simulink model "case8"  (R2024b)
settings: Solver=FixedStepAuto  StartTime=0  StopTime=1  FixedStep=1e-7  RelTol=1e-3
values from neighbouring files (symbols this model uses):
  SG_D_1_D = 0.01056    [IEEE9_case_parameters.m]    (also in case1_parameters.m; case2_parameters.m; case3_parameters.m; case4_parameters.m)
  SG_D_1_EnableSaturation = 0    [IEEE9_case_parameters.m]    (also in case1_parameters.m; case2_parameters.m; case3_parameters.m; case4_parameters.m)
  SG_D_1_f0 = 60    [IEEE9_case_parameters.m]    (also in case1_parameters.m; case2_parameters.m; case3_parameters.m; case4_parameters.m)
  SG_D_1_H = 7.5    [IEEE9_case_parameters.m]    (also in case1_parameters.m; case2_parameters.m; case3_parameters.m; case4_parameters.m)
  SG_D_1_K_A = 20    [IEEE9_case_parameters.m]    (also in case1_parameters.m; case2_parameters.m; case3_parameters.m; case4_parameters.m)
  SG_D_1_K_E = 1.000000e+1    (= 10)    [IEEE9_case_parameters.m]    (also in case1_parameters.m; case2_parameters.m; case3_parameters.m; case4_parameters.m)
  SG_D_1_K_F = 2.363    [IEEE9_case_parameters.m]    (also in case1_parameters.m; case2_parameters.m; case3_parameters.m; case4_parameters.m)
  SG_D_1_K_s = 0.5    [IEEE9_case_parameters.m]    (also in case1_parameters.m = 5; case2_parameters.m = 5; case3_parameters.m = 5; case4_parameters.m = 5)
  SG_D_1_R_a = 0.001088    [IEEE9_case_parameters.m]    (also in case1_parameters.m; case2_parameters.m; case3_parameters.m; case4_parameters.m)
  SG_D_1_S_A = 1    [IEEE9_case_parameters.m]    (also in case1_parameters.m; case2_parameters.m; case3_parameters.m; case4_parameters.m)
  SG_D_1_S_B = 0.103    [IEEE9_case_parameters.m]    (also in case1_parameters.m; case2_parameters.m; case3_parameters.m; case4_parameters.m)
  SG_D_1_S_N = 10.659857    [IEEE9_case_parameters.m]    (also in case1_parameters.m; case2_parameters.m; case3_parameters.m; case4_parameters.m)
  SG_D_1_SpeedPara = 200    [IEEE9_case_parameters.m]    (also in case1_parameters.m; case2_parameters.m; case3_parameters.m; case4_parameters.m)
  SG_D_1_T_0 = 0.720173    [IEEE9_case_parameters.m]    (also in case1_parameters.m = 0.755522; case2_parameters.m = 0.808931; case3_parameters.m = 0.869402; case4_parameters.m = 0.729316)
  SG_D_1_T_1 = 0.3    [IEEE9_case_parameters.m]    (also in case1_parameters.m; case2_parameters.m; case3_parameters.m; case4_parameters.m)
  SG_D_1_T_2 = 0.05    [IEEE9_case_parameters.m]    (also in case1_parameters.m; case2_parameters.m; case3_parameters.m; case4_parameters.m)
  SG_D_1_T_3 = 0.02    [IEEE9_case_parameters.m]    (also in case1_parameters.m; case2_parameters.m; case3_parameters.m; case4_parameters.m)
  SG_D_1_T_4 = 0.005    [IEEE9_case_parameters.m]    (also in case1_parameters.m; case2_parameters.m; case3_parameters.m; case4_parameters.m)
  SG_D_1_T_A = 0.02    [IEEE9_case_parameters.m]    (also in case1_parameters.m; case2_parameters.m; case3_parameters.m; case4_parameters.m)
  SG_D_1_T_dd = 8.000000e+0    (= 8)    [IEEE9_case_parameters.m]    (also in case1_parameters.m; case2_parameters.m; case3_parameters.m; case4_parameters.m)
  SG_D_1_T_ddd = 0.04    [IEEE9_case_parameters.m]    (also in case1_parameters.m; case2_parameters.m; case3_parameters.m; case4_parameters.m)
  SG_D_1_T_E = 0.314    [IEEE9_case_parameters.m]    (also in case1_parameters.m; case2_parameters.m; case3_parameters.m; case4_parameters.m)
  SG_D_1_T_F = 0.35    [IEEE9_case_parameters.m]    (also in case1_parameters.m; case2_parameters.m; case3_parameters.m; case4_parameters.m)
  SG_D_1_T_qd = 0.8    [IEEE9_case_parameters.m]    (also in case1_parameters.m; case2_parameters.m; case3_parameters.m; case4_parameters.m)
  SG_D_1_T_qdd = 0.02    [IEEE9_case_parameters.m]    (also in case1_parameters.m; case2_parameters.m; case3_parameters.m; case4_parameters.m)
  SG_D_1_T_speed = 0.1    [IEEE9_case_parameters.m]    (also in case1_parameters.m = 200; case2_parameters.m = 200; case3_parameters.m = 200; case4_parameters.m = 200)
  SG_D_1_T_w = 0.5    [IEEE9_case_parameters.m]    (also in case1_parameters.m; case2_parameters.m; case3_parameters.m; case4_parameters.m)
  SG_D_1_V_ref = 1.990276    [IEEE9_case_parameters.m]    (also in case1_parameters.m = 2.042296; case2_parameters.m = 2.051388; case3_parameters.m = 2.089584; case4_parameters.m = 2.01845)
  SG_D_1_w_ref = 376.991118    [IEEE9_case_parameters.m]    (also in case1_parameters.m; case2_parameters.m; case3_parameters.m; case4_parameters.m)
  SG_D_1_wb = 6.000000e+1    (= 60)    [IEEE9_case_parameters.m]    (also in case1_parameters.m; case2_parameters.m; case3_parameters.m; case4_parameters.m)
  SG_D_1_x_d = 1.9    [IEEE9_case_parameters.m]    (also in case1_parameters.m; case2_parameters.m; case3_parameters.m; case4_parameters.m)
  SG_D_1_x_dd = 0.302    [IEEE9_case_parameters.m]    (also in case1_parameters.m; case2_parameters.m; case3_parameters.m; case4_parameters.m)
  SG_D_1_x_ddd = 0.204    [IEEE9_case_parameters.m]    (also in case1_parameters.m; case2_parameters.m; case3_parameters.m; case4_parameters.m)
  SG_D_1_x_l = 0.05    [IEEE9_case_parameters.m]    (also in case1_parameters.m; case2_parameters.m; case3_parameters.m; case4_parameters.m)
  SG_D_1_x_q = 1.3    [IEEE9_case_parameters.m]    (also in case1_parameters.m; case2_parameters.m; case3_parameters.m; case4_parameters.m)
  SG_D_1_x_qd = 0.5    [IEEE9_case_parameters.m]    (also in case1_parameters.m; case2_parameters.m; case3_parameters.m; case4_parameters.m)
  SG_D_1_x_qdd = 0.3    [IEEE9_case_parameters.m]    (also in case1_parameters.m; case2_parameters.m; case3_parameters.m; case4_parameters.m)
  SG_D_2_D = 0.02    [IEEE9_case_parameters.m]    (also in case1_parameters.m; case2_parameters.m; case3_parameters.m; case4_parameters.m)
  SG_D_2_EnableSaturation = 0    [IEEE9_case_parameters.m]    (also in case1_parameters.m; case2_parameters.m; case3_parameters.m; case4_parameters.m)
  SG_D_2_f0 = 60    [IEEE9_case_parameters.m]    (also in case1_parameters.m; case2_parameters.m; case3_parameters.m; case4_parameters.m)
  SG_D_2_H = 8.000000e+0    (= 8)    [IEEE9_case_parameters.m]    (also in case1_parameters.m; case2_parameters.m; case3_parameters.m; case4_parameters.m)
  SG_D_2_K_A = 20    [IEEE9_case_parameters.m]    (also in case1_parameters.m; case2_parameters.m; case3_parameters.m; case4_parameters.m)
  SG_D_2_K_E = 1.000000e+1    (= 10)    [IEEE9_case_parameters.m]    (also in case1_parameters.m; case2_parameters.m; case3_parameters.m; case4_parameters.m)
  SG_D_2_K_F = 2.363    [IEEE9_case_parameters.m]    (also in case1_parameters.m; case2_parameters.m; case3_parameters.m; case4_parameters.m)
  SG_D_2_K_s = 0.5    [IEEE9_case_parameters.m]    (also in case1_parameters.m = 4; case2_parameters.m = 4; case3_parameters.m = 4; case4_parameters.m = 4)
  SG_D_2_R_a = 0.001088    [IEEE9_case_parameters.m]    (also in case1_parameters.m; case2_parameters.m; case3_parameters.m; case4_parameters.m)
  SG_D_2_S_A = 1    [IEEE9_case_parameters.m]    (also in case1_parameters.m; case2_parameters.m; case3_parameters.m; case4_parameters.m)
  SG_D_2_S_B = 0.103    [IEEE9_case_parameters.m]    (also in case1_parameters.m; case2_parameters.m; case3_parameters.m; case4_parameters.m)
  SG_D_2_S_N = 10.659857    [IEEE9_case_parameters.m]    (also in case1_parameters.m; case2_parameters.m; case3_parameters.m; case4_parameters.m)
  SG_D_2_SpeedPara = 200    [IEEE9_case_parameters.m]    (also in case1_parameters.m; case2_parameters.m; case3_parameters.m; case4_parameters.m)
  SG_D_2_T_0 = 1.632913    [IEEE9_case_parameters.m]    (also in case1_parameters.m = 1.632925; case2_parameters.m = 1.632915; case3_parameters.m = 1.632914; case4_parameters.m = 1.632927)
  SG_D_2_T_1 = 0.2    [IEEE9_case_parameters.m]    (also in case1_parameters.m; case2_parameters.m; case3_parameters.m; case4_parameters.m)
  SG_D_2_T_2 = 0.05    [IEEE9_case_parameters.m]    (also in case1_parameters.m; case2_parameters.m; case3_parameters.m; case4_parameters.m)
  SG_D_2_T_3 = 0.02    [IEEE9_case_parameters.m]    (also in case1_parameters.m; case2_parameters.m; case3_parameters.m; case4_parameters.m)
  SG_D_2_T_4 = 0.005    [IEEE9_case_parameters.m]    (also in case1_parameters.m; case2_parameters.m; case3_parameters.m; case4_parameters.m)
  SG_D_2_T_A = 0.02    [IEEE9_case_parameters.m]    (also in case1_parameters.m; case2_parameters.m; case3_parameters.m; case4_parameters.m)
  SG_D_2_T_dd = 7.9    [IEEE9_case_parameters.m]    (also in case1_parameters.m; case2_parameters.m; case3_parameters.m; case4_parameters.m)
  SG_D_2_T_ddd = 0.04    [IEEE9_case_parameters.m]    (also in case1_parameters.m; case2_parameters.m; case3_parameters.m; case4_parameters.m)
  SG_D_2_T_E = 0.314    [IEEE9_case_parameters.m]    (also in case1_parameters.m; case2_parameters.m; case3_parameters.m; case4_parameters.m)
  SG_D_2_T_F = 0.35    [IEEE9_case_parameters.m]    (also in case1_parameters.m; case2_parameters.m; case3_parameters.m; case4_parameters.m)
  SG_D_2_T_qd = 0.8    [IEEE9_case_parameters.m]    (also in case1_parameters.m; case2_parameters.m; case3_parameters.m; case4_parameters.m)
  SG_D_2_T_qdd = 0.015    [IEEE9_case_parameters.m]    (also in case1_parameters.m; case2_parameters.m; case3_parameters.m; case4_parameters.m)
  SG_D_2_T_speed = 0.1    [IEEE9_case_parameters.m]    (also in case1_parameters.m = 150; case2_parameters.m = 150; case3_parameters.m = 150; case4_parameters.m = 150)
  SG_D_2_T_w = 0.35    [IEEE9_case_parameters.m]    (also in case1_parameters.m; case2_parameters.m; case3_parameters.m; case4_parameters.m)
  SG_D_2_V_ref = 2.58547    [IEEE9_case_parameters.m]    (also in case1_parameters.m = 2.597896; case2_parameters.m = 2.587136; case3_parameters.m = 2.586042; case4_parameters.m = 2.599679)
  SG_D_2_w_ref = 376.991118    [IEEE9_case_parameters.m]    (also in case1_parameters.m; case2_parameters.m; case3_parameters.m; case4_parameters.m)
  SG_D_2_wb = 6.000000e+1    (= 60)    [IEEE9_case_parameters.m]    (also in case1_parameters.m; case2_parameters.m; case3_parameters.m; case4_parameters.m)
  SG_D_2_x_d = 1.8    [IEEE9_case_parameters.m]    (also in case1_parameters.m; case2_parameters.m; case3_parameters.m; case4_parameters.m)
  SG_D_2_x_dd = 0.302    [IEEE9_case_parameters.m]    (also in case1_parameters.m; case2_parameters.m; case3_parameters.m; case4_parameters.m)
  SG_D_2_x_ddd = 0.204    [IEEE9_case_parameters.m]    (also in case1_parameters.m; case2_parameters.m; case3_parameters.m; case4_parameters.m)
  SG_D_2_x_l = 0.05    [IEEE9_case_parameters.m]    (also in case1_parameters.m; case2_parameters.m; case3_parameters.m; case4_parameters.m)
  SG_D_2_x_q = 1.25    [IEEE9_case_parameters.m]    (also in case1_parameters.m; case2_parameters.m; case3_parameters.m; case4_parameters.m)
  SG_D_2_x_qd = 0.5    [IEEE9_case_parameters.m]    (also in case1_parameters.m; case2_parameters.m; case3_parameters.m; case4_parameters.m)
  SG_D_2_x_qdd = 0.3    [IEEE9_case_parameters.m]    (also in case1_parameters.m; case2_parameters.m; case3_parameters.m; case4_parameters.m)
  SG_D_3_D = 0.02    [IEEE9_case_parameters.m]    (also in case1_parameters.m; case2_parameters.m; case3_parameters.m; case4_parameters.m)
  SG_D_3_EnableSaturation = 0    [IEEE9_case_parameters.m]    (also in case1_parameters.m; case2_parameters.m; case3_parameters.m; case4_parameters.m)
  SG_D_3_f0 = 60    [IEEE9_case_parameters.m]    (also in case1_parameters.m; case2_parameters.m; case3_parameters.m; case4_parameters.m)
  SG_D_3_H = 7.7    [IEEE9_case_parameters.m]    (also in case1_parameters.m; case2_parameters.m; case3_parameters.m; case4_parameters.m)
  SG_D_3_K_A = 20    [IEEE9_case_parameters.m]    (also in case1_parameters.m; case2_parameters.m; case3_parameters.m; case4_parameters.m)
  SG_D_3_K_E = 1.000000e+1    (= 10)    [IEEE9_case_parameters.m]    (also in case1_parameters.m; case2_parameters.m; case3_parameters.m; case4_parameters.m)
  SG_D_3_K_F = 2.363    [IEEE9_case_parameters.m]    (also in case1_parameters.m; case2_parameters.m; case3_parameters.m; case4_parameters.m)
  SG_D_3_K_s = 0.2    [IEEE9_case_parameters.m]    (also in case1_parameters.m = 2; case2_parameters.m = 2; case3_parameters.m = 2; case4_parameters.m = 2)
  SG_D_3_R_a = 0.001088    [IEEE9_case_parameters.m]    (also in case1_parameters.m; case2_parameters.m; case3_parameters.m; case4_parameters.m)
  SG_D_3_S_A = 1    [IEEE9_case_parameters.m]    (also in case1_parameters.m; case2_parameters.m; case3_parameters.m; case4_parameters.m)
  SG_D_3_S_B = 0.103    [IEEE9_case_parameters.m]    (also in case1_parameters.m; case2_parameters.m; case3_parameters.m; case4_parameters.m)
  SG_D_3_S_N = 10.659857    [IEEE9_case_parameters.m]    (also in case1_parameters.m; case2_parameters.m; case3_parameters.m; case4_parameters.m)
  SG_D_3_SpeedPara = 200    [IEEE9_case_parameters.m]    (also in case1_parameters.m; case2_parameters.m; case3_parameters.m; case4_parameters.m)
  SG_D_3_T_0 = 0.850788    [IEEE9_case_parameters.m]    (also in case1_parameters.m = 0.850786; case2_parameters.m = 0.850787; case3_parameters.m; case4_parameters.m = 0.850786)
  SG_D_3_T_1 = 0.2    [IEEE9_case_parameters.m]    (also in case1_parameters.m; case2_parameters.m; case3_parameters.m; case4_parameters.m)
  SG_D_3_T_2 = 0.05    [IEEE9_case_parameters.m]    (also in case1_parameters.m; case2_parameters.m; case3_parameters.m; case4_parameters.m)
  SG_D_3_T_3 = 0.02    [IEEE9_case_parameters.m]    (also in case1_parameters.m; case2_parameters.m; case3_parameters.m; case4_parameters.m)
  SG_D_3_T_4 = 0.005    [IEEE9_case_parameters.m]    (also in case1_parameters.m; case2_parameters.m; case3_parameters.m; case4_parameters.m)
  SG_D_3_T_A = 0.02    [IEEE9_case_parameters.m]    (also in case1_parameters.m; case2_parameters.m; case3_parameters.m; case4_parameters.m)
  SG_D_3_T_dd = 8.1    [IEEE9_case_parameters.m]    (also in case1_parameters.m; case2_parameters.m; case3_parameters.m; case4_parameters.m)
  SG_D_3_T_ddd = 0.04    [IEEE9_case_parameters.m]    (also in case1_parameters.m; case2_parameters.m; case3_parameters.m; case4_parameters.m)
  SG_D_3_T_E = 0.314    [IEEE9_case_parameters.m]    (also in case1_parameters.m; case2_parameters.m; case3_parameters.m; case4_parameters.m)
  SG_D_3_T_F = 0.35    [IEEE9_case_parameters.m]    (also in case1_parameters.m; case2_parameters.m; case3_parameters.m; case4_parameters.m)
  SG_D_3_T_qd = 0.8    [IEEE9_case_parameters.m]    (also in case1_parameters.m; case2_parameters.m; case3_parameters.m; case4_parameters.m)
  SG_D_3_T_qdd = 0.015    [IEEE9_case_parameters.m]    (also in case1_parameters.m; case2_parameters.m; case3_parameters.m; case4_parameters.m)
  SG_D_3_T_speed = 0.1    [IEEE9_case_parameters.m]    (also in case1_parameters.m = 180; case2_parameters.m = 180; case3_parameters.m = 180; case4_parameters.m = 180)
  SG_D_3_T_w = 0.4    [IEEE9_case_parameters.m]    (also in case1_parameters.m; case2_parameters.m; case3_parameters.m; case4_parameters.m)
  SG_D_3_V_ref = 1.892727    [IEEE9_case_parameters.m]    (also in case1_parameters.m = 1.906439; case2_parameters.m = 1.895535; case3_parameters.m = 1.892105; case4_parameters.m = 1.906598)
  SG_D_3_w_ref = 376.991118    [IEEE9_case_parameters.m]    (also in case1_parameters.m; case2_parameters.m; case3_parameters.m; case4_parameters.m)
  SG_D_3_wb = 6.000000e+1    (= 60)    [IEEE9_case_parameters.m]    (also in case1_parameters.m; case2_parameters.m; case3_parameters.m; case4_parameters.m)
  SG_D_3_x_d = 1.85    [IEEE9_case_parameters.m]    (also in case1_parameters.m; case2_parameters.m; case3_parameters.m; case4_parameters.m)
  SG_D_3_x_dd = 0.302    [IEEE9_case_parameters.m]    (also in case1_parameters.m; case2_parameters.m; case3_parameters.m; case4_parameters.m)
  SG_D_3_x_ddd = 0.204    [IEEE9_case_parameters.m]    (also in case1_parameters.m; case2_parameters.m; case3_parameters.m; case4_parameters.m)
  SG_D_3_x_l = 0.05    [IEEE9_case_parameters.m]    (also in case1_parameters.m; case2_parameters.m; case3_parameters.m; case4_parameters.m)
  SG_D_3_x_q = 1.2    [IEEE9_case_parameters.m]    (also in case1_parameters.m; case2_parameters.m; case3_parameters.m; case4_parameters.m)
  SG_D_3_x_qd = 0.5    [IEEE9_case_parameters.m]    (also in case1_parameters.m; case2_parameters.m; case3_parameters.m; case4_parameters.m)
  SG_D_3_x_qdd = 0.3    [IEEE9_case_parameters.m]    (also in case1_parameters.m; case2_parameters.m; case3_parameters.m; case4_parameters.m)
(part 8 of 12)

== system case8/SG_D_2/d_psi_d_SG_D_2_block ==
  note: d_psi_d_SG_D_2 in case8
      | $2\,\pi \,f_{0}\,\left(v_{d,\mathrm{SG},D,2}\,\sin\left(\theta _{\mathrm{SG},D,2}\right)-v_{q,\mathrm{SG},D,2}\,\cos\left(\theta _{\mathrm{SG},D,2}\right)+\frac{R_{a}\,\left(\frac{\psi _{\mathrm{1d},\mathrm{SG},D,2}\,\left(x_{\mathrm{dd}}-x_{\mathrm{ddd}}\right)}{x_{\mathrm{dd}}-x_{l}}-\psi _{d,\mathrm{SG},D,2}+\frac{\psi _{\mathrm{fd},\mathrm{SG},D,2}\,\left(x_{\mathrm{ddd}}-x_{l}\right)}{x_{\mathrm{dd}}-x_{l}}\right)}{x_{\mathrm{ddd}}}+\frac{\psi _{q,\mathrm{SG},D,2}\,w_{\mathrm{SG},D,2}}{2\,f_{0}\,\pi }\right)$
      | Automatically generated on 2025-10-31 19:29:46 .
  State_psi_1d_SG_D_2_aad77 : Inport
  State_psi_d_SG_D_2_6f046 : Inport  Port=2
  State_psi_fd_SG_D_2_72f19 : Inport  Port=3
  Input_v_d_SG_D_2_0b52f : Inport  Port=4
  State_theta_SG_D_2_93d8b : Inport  Port=5
  Input_v_q_SG_D_2_24264 : Inport  Port=6
  State_theta_SG_D_2_1c678 : Inport  Port=7
  State_psi_q_SG_D_2_6ca96 : Inport  Port=8
  State_w_SG_D_2_45274 : Inport  Port=9
  Add_49bc6 : Sum
  Add_4ccb7 : Sum
  Constant_-1_a1881 : Constant  Value=-1
  Constant_-2.0_16ca3 : Constant  Value=-2.0
  Constant_2.0_65f11 : Constant  Value=2.0
  Constant_R_a_a2532 : Constant  Value=R_a
  Constant_f0_5dad4 : Constant  Value=f0
  Constant_f0_a6411 : Constant  Value=f0
  Constant_pi_112bc : Constant  Value=pi
  Constant_pi_f3391 : Constant  Value=pi
  Constant_x_dd_02a07 : Constant  Value=x_dd
  Constant_x_dd_564c6 : Constant  Value=x_dd
  Constant_x_dd_64ecc : Constant  Value=x_dd
  Constant_x_ddd_3802c : Constant  Value=x_ddd
  Constant_x_ddd_72880 : Constant  Value=x_ddd
  Constant_x_ddd_8e95c : Constant  Value=x_ddd
  Constant_x_l_5badf : Constant  Value=x_l
  Constant_x_l_a4c95 : Constant  Value=x_l
  Constant_x_l_b061f : Constant  Value=x_l
  Divide_41e9e : Product  Inputs=*/
  Divide_5bfee : Product  Inputs=*/
  Divide_6ddcf : Product  Inputs=*/
  Divide_cf75d : Product  Inputs=*/
  MathFunc_cos_91622 : Trigonometry  Operator=cos
  MathFunc_sin_e79ab : Trigonometry
  Product_13311 : Product
  Product_54dec : Product
  Product_5e8bb : Product
  Product_74e91 : Product
  Product_981a3 : Product
  Product_a6b38 : Product
  Product_a97df : Product
  Product_b3f10 : Product
  Product_b96ae : Product
  Product_d093f : Product
  Product_ee3a2 : Product
  Product_f3a68 : Product
  Subtract_16af1 : Sum  Inputs=+-
  Subtract_1704f : Sum  Inputs=+-
  Subtract_8b765 : Sum  Inputs=+-
  Subtract_a1fd3 : Sum  Inputs=+-
  Subtract_c9d0d : Sum  Inputs=+-
  Subtract_cea0f : Sum  Inputs=+-
  Subtract_d5c02 : Sum  Inputs=+-
  Blockout_d_psi_d_SG_D_2_41311 : Outport
  wires:
  MathFunc_sin_e79ab/1 -> Product_74e91/2
  Constant_x_dd_564c6/1 -> Subtract_16af1/1
  Constant_-1_a1881/1 -> Product_981a3/1
  Constant_x_l_5badf/1 -> Subtract_16af1/2
  State_psi_1d_SG_D_2_aad77/1 -> Product_981a3/2
  Constant_f0_5dad4/1 -> Product_ee3a2/2
  Constant_2.0_65f11/1 -> Product_54dec/1
  Constant_x_l_a4c95/1 -> Subtract_cea0f/2
  Constant_x_dd_64ecc/1 -> Subtract_c9d0d/1
  Product_a6b38/1 -> Blockout_d_psi_d_SG_D_2_41311/1
  Constant_pi_f3391/1 -> Product_54dec/2
  Constant_x_ddd_3802c/1 -> Subtract_c9d0d/2
  Subtract_1704f/1 -> Product_a6b38/2
  Product_981a3/1 -> Product_b3f10/1
  Product_54dec/1 -> Product_13311/1
  Subtract_c9d0d/1 -> Product_b3f10/2
  Divide_41e9e/1 -> Subtract_1704f/2
  Constant_x_ddd_72880/1 -> Subtract_a1fd3/1
  Constant_x_l_b061f/1 -> Subtract_a1fd3/2
  Product_b3f10/1 -> Divide_cf75d/1
  Subtract_8b765/1 -> Add_4ccb7/1
  Subtract_16af1/1 -> Divide_cf75d/2
  State_psi_fd_SG_D_2_72f19/1 -> Product_5e8bb/1
  Subtract_a1fd3/1 -> Product_5e8bb/2
  Constant_x_dd_02a07/1 -> Subtract_cea0f/1
  Divide_cf75d/1 -> Add_49bc6/1
  State_psi_d_SG_D_2_6f046/1 -> Add_49bc6/2
  Product_5e8bb/1 -> Divide_6ddcf/1
  Subtract_cea0f/1 -> Divide_6ddcf/2
  Add_49bc6/1 -> Subtract_d5c02/1
  Divide_6ddcf/1 -> Subtract_d5c02/2
  Constant_R_a_a2532/1 -> Product_f3a68/1
  Subtract_d5c02/1 -> Product_f3a68/2
  Divide_5bfee/1 -> Subtract_8b765/1
  State_theta_SG_D_2_93d8b/1 -> MathFunc_sin_e79ab/1
  Product_f3a68/1 -> Divide_5bfee/1
  Constant_-2.0_16ca3/1 -> Product_b96ae/1
  Input_v_d_SG_D_2_0b52f/1 -> Product_74e91/1
  Constant_x_ddd_8e95c/1 -> Divide_5bfee/2
  State_theta_SG_D_2_1c678/1 -> MathFunc_cos_91622/1
  Product_ee3a2/1 -> Product_a6b38/1
  Product_74e91/1 -> Subtract_8b765/2
  Product_b96ae/1 -> Product_ee3a2/1
  Input_v_q_SG_D_2_24264/1 -> Product_d093f/1
  MathFunc_cos_91622/1 -> Product_d093f/2
  State_psi_q_SG_D_2_6ca96/1 -> Product_a97df/1
  State_w_SG_D_2_45274/1 -> Product_a97df/2
  Constant_f0_a6411/1 -> Product_13311/2
  Constant_pi_112bc/1 -> Product_b96ae/2
  Product_d093f/1 -> Add_4ccb7/2
  Product_a97df/1 -> Divide_41e9e/1
  Product_13311/1 -> Divide_41e9e/2
  Add_4ccb7/1 -> Subtract_1704f/1

== system case8/SG_D_2/d_psi_fd_SG_D_2_block ==
  note: d_psi_fd_SG_D_2 in case8
      | $-\frac{\psi _{\mathrm{fd},\mathrm{SG},D,2}-E_{\mathrm{fd},\mathrm{SG},D,2}+\left(x_{d}-x_{\mathrm{dd}}\right)\,\left(\frac{\frac{\psi _{\mathrm{1d},\mathrm{SG},D,2}\,\left(x_{\mathrm{dd}}-x_{\mathrm{ddd}}\right)}{x_{\mathrm{dd}}-x_{l}}-\psi _{d,\mathrm{SG},D,2}+\frac{\psi _{\mathrm{fd},\mathrm{SG},D,2}\,\left(x_{\mathrm{ddd}}-x_{l}\right)}{x_{\mathrm{dd}}-x_{l}}}{x_{\mathrm{ddd}}}-\frac{\left(x_{\mathrm{dd}}-x_{\mathrm{ddd}}\right)\,\left(\psi _{\mathrm{1d},\mathrm{SG},D,2}-\psi _{\mathrm{fd},\mathrm{SG},D,2}+\frac{\left(x_{\mathrm{dd}}-x_{l}\right)\,\left(\frac{\psi _{\mathrm{1d},\mathrm{SG},D,2}\,\left(x_{\mathrm{dd}}-x_{\mathrm{ddd}}\right)}{x_{\mathrm{dd}}-x_{l}}-\psi _{d,\mathrm{SG},D,2}+\frac{\psi _{\mathrm{fd},\mathrm{SG},D,2}\,\left(x_{\mathrm{ddd}}-x_{l}\right)}{x_{\mathrm{dd}}-x_{l}}\right)}{x_{\mathrm{ddd}}}\right)}{{\left(x_{\mathrm{dd}}-x_{l}\right)}^2}\right)}{T_{\mathrm{dd}}}$
      | Automatically generated on 2025-10-31 19:29:48 .
  State_E_fd_SG_D_2_e61ef : Inport
  State_psi_fd_SG_D_2_b4c0c : Inport  Port=2
  State_psi_1d_SG_D_2_30ef8 : Inport  Port=3
  State_psi_fd_SG_D_2_4158a : Inport  Port=4
  State_psi_1d_SG_D_2_923e8 : Inport  Port=5
  State_psi_d_SG_D_2_db85c : Inport  Port=6
  State_psi_fd_SG_D_2_07a98 : Inport  Port=7
  State_psi_1d_SG_D_2_d512d : Inport  Port=8
  State_psi_d_SG_D_2_0ff1e : Inport  Port=9
  State_psi_fd_SG_D_2_1b762 : Inport  Port=10
  Add_5a7e8 : Sum
  Add_f1187 : Sum
  Constant_-1_837ce : Constant  Value=-1
  Constant_-1_c4842 : Constant  Value=-1
  Constant_-1_e6265 : Constant  Value=-1
  Constant_2.0_bbcc8 : Constant  Value=2.0
  Constant_T_dd_00900 : Constant  Value=T_dd
  Constant_x_d_c7ce0 : Constant  Value=x_d
  Constant_x_dd_351c8 : Constant  Value=x_dd
  Constant_x_dd_4b32a : Constant  Value=x_dd
  Constant_x_dd_4d4b9 : Constant  Value=x_dd
  Constant_x_dd_500db : Constant  Value=x_dd
  Constant_x_dd_5326d : Constant  Value=x_dd
  Constant_x_dd_592f2 : Constant  Value=x_dd
  Constant_x_dd_7b2bb : Constant  Value=x_dd
  Constant_x_dd_85d34 : Constant  Value=x_dd
  Constant_x_dd_d530f : Constant  Value=x_dd
  Constant_x_dd_d5f8d : Constant  Value=x_dd
  Constant_x_ddd_43065 : Constant  Value=x_ddd
  Constant_x_ddd_5fbd9 : Constant  Value=x_ddd
  Constant_x_ddd_b579f : Constant  Value=x_ddd
  Constant_x_ddd_c5a8f : Constant  Value=x_ddd
  Constant_x_ddd_d7223 : Constant  Value=x_ddd
  Constant_x_ddd_dfbab : Constant  Value=x_ddd
  Constant_x_ddd_e8f08 : Constant  Value=x_ddd
  Constant_x_l_428fa : Constant  Value=x_l
  Constant_x_l_47188 : Constant  Value=x_l
  Constant_x_l_5d447 : Constant  Value=x_l
  Constant_x_l_72a37 : Constant  Value=x_l
  Constant_x_l_74678 : Constant  Value=x_l
  Constant_x_l_aa512 : Constant  Value=x_l
  Constant_x_l_cff61 : Constant  Value=x_l
  Constant_x_l_fd167 : Constant  Value=x_l
  Divide_19e00 : Product  Inputs=*/
  Divide_1cd42 : Product  Inputs=*/
  Divide_36d83 : Product  Inputs=*/
  Divide_425e5 : Product  Inputs=*/
  Divide_537c9 : Product  Inputs=*/
  Divide_77337 : Product  Inputs=*/
  Divide_9c0b3 : Product  Inputs=*/
  Divide_ac56c : Product  Inputs=*/
  Power_8b02d : Math  Operator=pow
  Product_0bca5 : Product
  Product_19410 : Product
  Product_32052 : Product
  Product_4f906 : Product
  Product_5f94a : Product
  Product_76df1 : Product
  Product_a6bc6 : Product
  Product_b1a03 : Product
  Product_d6388 : Product
  Product_fabcd : Product
  Subtract_021aa : Sum  Inputs=+-
  Subtract_0b5a2 : Sum  Inputs=+-
  Subtract_0d3c1 : Sum  Inputs=+-
  Subtract_22515 : Sum  Inputs=+-
  Subtract_2a3bd : Sum  Inputs=+-
  Subtract_411a7 : Sum  Inputs=+-
  Subtract_4a648 : Sum  Inputs=+-
  Subtract_572ac : Sum  Inputs=+-
  Subtract_59e44 : Sum  Inputs=+-
  Subtract_6013b : Sum  Inputs=+-
  Subtract_73638 : Sum  Inputs=+-
  Subtract_785ab : Sum  Inputs=+-
  Subtract_80700 : Sum  Inputs=+-
  Subtract_99ee6 : Sum  Inputs=+-
  Subtract_be581 : Sum  Inputs=+-
  Subtract_bf9ce : Sum  Inputs=+-
  Subtract_d618a : Sum  Inputs=+-
  Subtract_ec7b4 : Sum  Inputs=+-
  Subtract_f94ca : Sum  Inputs=+-
  Blockout_d_psi_fd_SG_D_2_e5dbf : Outport
  wires:
  Constant_x_dd_4d4b9/1 -> Subtract_59e44/1
  Constant_-1_837ce/1 -> Product_fabcd/1
  Constant_x_l_72a37/1 -> Subtract_80700/2
  Divide_1cd42/1 -> Add_5a7e8/1
  Subtract_2a3bd/1 -> Product_32052/2
  Constant_x_l_fd167/1 -> Subtract_59e44/2
  Product_32052/1 -> Divide_ac56c/1
  State_psi_1d_SG_D_2_923e8/1 -> Product_fabcd/2
  Constant_x_dd_500db/1 -> Subtract_021aa/1
  Product_76df1/1 -> Divide_1cd42/1
  Constant_x_dd_d5f8d/1 -> Subtract_d618a/1
  Constant_x_ddd_c5a8f/1 -> Subtract_021aa/2
  Constant_x_dd_d530f/1 -> Subtract_0d3c1/1
  Product_fabcd/1 -> Product_5f94a/1
  Subtract_021aa/1 -> Product_5f94a/2
  State_psi_d_SG_D_2_0ff1e/1 -> Add_5a7e8/2
  Constant_x_ddd_5fbd9/1 -> Subtract_2a3bd/1
  Constant_x_l_cff61/1 -> Subtract_2a3bd/2
  Product_5f94a/1 -> Divide_77337/1
  Subtract_59e44/1 -> Divide_77337/2
  State_psi_fd_SG_D_2_07a98/1 -> Product_32052/1
  Subtract_22515/1 -> Product_b1a03/2
  Constant_x_dd_592f2/1 -> Subtract_411a7/1
  Constant_x_l_47188/1 -> Subtract_411a7/2
  Product_a6bc6/1 -> Product_b1a03/1
  Divide_77337/1 -> Add_f1187/1
  State_psi_d_SG_D_2_db85c/1 -> Add_f1187/2
  Subtract_411a7/1 -> Divide_ac56c/2
  Constant_x_dd_4b32a/1 -> Subtract_80700/1
  Constant_x_ddd_dfbab/1 -> Subtract_6013b/1
  Add_f1187/1 -> Subtract_785ab/1
  Divide_ac56c/1 -> Subtract_785ab/2
  Constant_-1_e6265/1 -> Product_d6388/1
  Product_19410/1 -> Divide_537c9/1
  State_psi_1d_SG_D_2_d512d/1 -> Product_d6388/2
  Subtract_d618a/1 -> Product_a6bc6/2
  Constant_x_dd_5326d/1 -> Subtract_99ee6/1
  Divide_537c9/1 -> Subtract_572ac/2
  Constant_-1_c4842/1 -> Product_a6bc6/1
  Constant_x_ddd_e8f08/1 -> Subtract_99ee6/2
  Constant_x_ddd_b579f/1 -> Divide_36d83/2
  Subtract_80700/1 -> Product_0bca5/1
  Subtract_785ab/1 -> Product_0bca5/2
  State_psi_fd_SG_D_2_4158a/1 -> Subtract_73638/2
  Product_d6388/1 -> Product_76df1/1
  Subtract_99ee6/1 -> Product_76df1/2
  Constant_2.0_bbcc8/1 -> Power_8b02d/2
  State_psi_1d_SG_D_2_30ef8/1 -> Subtract_73638/1
  Constant_x_dd_351c8/1 -> Subtract_4a648/1
  Subtract_6013b/1 -> Product_19410/2
  Constant_x_l_428fa/1 -> Subtract_4a648/2
  Constant_x_l_5d447/1 -> Subtract_6013b/2
  Constant_x_ddd_d7223/1 -> Subtract_d618a/2
  Subtract_0d3c1/1 -> Divide_537c9/2
  Product_0bca5/1 -> Divide_36d83/1
  Subtract_4a648/1 -> Divide_1cd42/2
  State_psi_fd_SG_D_2_1b762/1 -> Product_19410/1
  Constant_x_l_aa512/1 -> Subtract_0d3c1/2
  Constant_x_dd_85d34/1 -> Subtract_ec7b4/1
  Subtract_73638/1 -> Subtract_22515/1
  Divide_36d83/1 -> Subtract_22515/2
  Constant_x_l_74678/1 -> Subtract_ec7b4/2
  Subtract_ec7b4/1 -> Power_8b02d/1
  Add_5a7e8/1 -> Subtract_572ac/1
  Product_b1a03/1 -> Divide_19e00/1
  Power_8b02d/1 -> Divide_19e00/2
  Subtract_572ac/1 -> Divide_425e5/1
  Constant_x_ddd_43065/1 -> Divide_425e5/2
  Constant_x_d_c7ce0/1 -> Subtract_f94ca/1
  Constant_x_dd_7b2bb/1 -> Subtract_f94ca/2
  Divide_19e00/1 -> Subtract_be581/1
  Divide_425e5/1 -> Subtract_be581/2
  State_E_fd_SG_D_2_e61ef/1 -> Subtract_0b5a2/1
  State_psi_fd_SG_D_2_b4c0c/1 -> Subtract_0b5a2/2
  Subtract_f94ca/1 -> Product_4f906/1
  Subtract_be581/1 -> Product_4f906/2
  Subtract_0b5a2/1 -> Subtract_bf9ce/1
  Product_4f906/1 -> Subtract_bf9ce/2
  Subtract_bf9ce/1 -> Divide_9c0b3/1
  Constant_T_dd_00900/1 -> Divide_9c0b3/2
  Divide_9c0b3/1 -> Blockout_d_psi_fd_SG_D_2_e5dbf/1

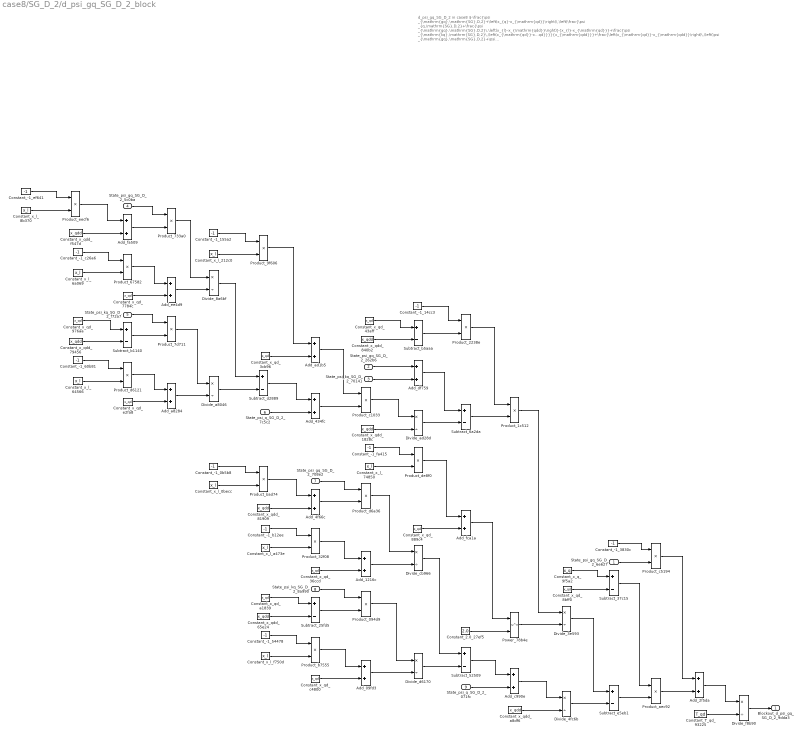
== system case8/SG_D_2/d_psi_gq_SG_D_2_block ==
  note: d_psi_gq_SG_D_2 in case8
      | $-\frac{\psi _{\mathrm{gq},\mathrm{SG},D,2}+\left(x_{q}-x_{\mathrm{qd}}\right)\,\left(\frac{\psi _{q,\mathrm{SG},D,2}+\frac{\psi _{\mathrm{gq},\mathrm{SG},D,2}\,\left(x_{l}-x_{\mathrm{qdd}}\right)}{x_{l}-x_{\mathrm{qd}}}+\frac{\psi _{\mathrm{kq},\mathrm{SG},D,2}\,\left(x_{\mathrm{qd}}-x_{\mathrm{qdd}}\right)}{x_{l}-x_{\mathrm{qd}}}}{x_{\mathrm{qdd}}}+\frac{\left(x_{\mathrm{qd}}-x_{\mathrm{qdd}}\right)\,\left(\psi _{\mathrm{gq},\mathrm{SG},D,2}+\psi _{\mathrm{kq},\mathrm{SG},D,2}+\frac{\left(x_{l}-x_{\mathrm{qd}}\right)\,\left(\psi _{q,\mathrm{SG},D,2}+\frac{\psi _{\mathrm{gq},\mathrm{SG},D,2}\,\left(x_{l}-x_{\mathrm{qdd}}\right)}{x_{l}-x_{\mathrm{qd}}}+\frac{\psi _{\mathrm{kq},\mathrm{SG},D,2}\,\left(x_{\mathrm{qd}}-x_{\mathrm{qdd}}\right)}{x_{l}-x_{\mathrm{qd}}}\right)}{x_{\mathrm{qdd}}}\right)}{{\left(x_{l}-x_{\mathrm{qd}}\right)}^2}\right)}{T_{\mathrm{qd}}}$
      | Automatically generated on 2025-10-31 19:29:51 .
  State_psi_gq_SG_D_2_6e627 : Inport
  State_psi_gq_SG_D_2_262b6 : Inport  Port=2
  State_psi_kq_SG_D_2_70141 : Inport  Port=3
  State_psi_gq_SG_D_2_5c0ba : Inport  Port=4
  State_psi_kq_SG_D_2_f72a7 : Inport  Port=5
  State_psi_q_SG_D_2_7c5c2 : Inport  Port=6
  State_psi_gq_SG_D_2_708e2 : Inport  Port=7
  State_psi_kq_SG_D_2_8a990 : Inport  Port=8
  State_psi_q_SG_D_2_071fc : Inport  Port=9
  Add_09fd3 : Sum
  Add_1216c : Sum
  Add_2f5da : Sum
  Add_434fc : Sum
  Add_4f66c : Sum
  Add_a8284 : Sum
  Add_ad1b5 : Sum
  Add_c990e : Sum
  Add_df759 : Sum
  Add_ee4d9 : Sum
  Add_fa509 : Sum
  Add_fca1a : Sum
  Constant_-1_0b5b8 : Constant  Value=-1
  Constant_-1_14cc3 : Constant  Value=-1
  Constant_-1_155a2 : Constant  Value=-1
  Constant_-1_3830c : Constant  Value=-1
  Constant_-1_54478 : Constant  Value=-1
  Constant_-1_60b81 : Constant  Value=-1
  Constant_-1_b12ee : Constant  Value=-1
  Constant_-1_c26a6 : Constant  Value=-1
  Constant_-1_ef641 : Constant  Value=-1
  Constant_-1_fa415 : Constant  Value=-1
  Constant_2.0_27ef5 : Constant  Value=2.0
  Constant_T_qd_93225 : Constant  Value=T_qd
  Constant_x_l_0becc : Constant  Value=x_l
  Constant_x_l_212c0 : Constant  Value=x_l
  Constant_x_l_64566 : Constant  Value=x_l
  Constant_x_l_6a069 : Constant  Value=x_l
  Constant_x_l_74850 : Constant  Value=x_l
  Constant_x_l_8b370 : Constant  Value=x_l
  Constant_x_l_a473e : Constant  Value=x_l
  Constant_x_l_f750d : Constant  Value=x_l
  Constant_x_q_9f5a2 : Constant  Value=x_q
  Constant_x_qd_36ccd : Constant  Value=x_qd
  Constant_x_qd_3cb96 : Constant  Value=x_qd
  Constant_x_qd_43aff : Constant  Value=x_qd
  Constant_x_qd_7784c : Constant  Value=x_qd
  Constant_x_qd_889c4 : Constant  Value=x_qd
  Constant_x_qd_8bff0 : Constant  Value=x_qd
  Constant_x_qd_976aa : Constant  Value=x_qd
  Constant_x_qd_a1839 : Constant  Value=x_qd
  Constant_x_qd_c4800 : Constant  Value=x_qd
  Constant_x_qd_e2fa8 : Constant  Value=x_qd
  Constant_x_qdd_1828c : Constant  Value=x_qdd
  Constant_x_qdd_65e24 : Constant  Value=x_qdd
  Constant_x_qdd_79456 : Constant  Value=x_qdd
  Constant_x_qdd_81909 : Constant  Value=x_qdd
  Constant_x_qdd_840b2 : Constant  Value=x_qdd
  Constant_x_qdd_a8df6 : Constant  Value=x_qdd
  Constant_x_qdd_f547d : Constant  Value=x_qdd
  Divide_3e593 : Product  Inputs=*/
  Divide_4fc6b : Product  Inputs=*/
  Divide_8a6bf : Product  Inputs=*/
  Divide_a8046 : Product  Inputs=*/
  Divide_ad28d : Product  Inputs=*/
  Divide_cb966 : Product  Inputs=*/
  Divide_d6170 : Product  Inputs=*/
  Divide_f8b90 : Product  Inputs=*/
  Power_78b4e : Math  Operator=pow
  Product_094d9 : Product
  Product_1c512 : Product
  Product_2238e : Product
  Product_32f08 : Product
  Product_67582 : Product
  Product_733a0 : Product
  Product_7d711 : Product
  Product_9f606 : Product
  Product_aec92 : Product
  Product_b7555 : Product
  Product_bad74 : Product
  Product_c1033 : Product
  Product_c5194 : Product
  Product_d6121 : Product
  Product_d6a36 : Product
  Product_de8f0 : Product
  Product_eecf6 : Product
  Subtract_25fd5 : Sum  Inputs=+-
  Subtract_37c15 : Sum  Inputs=+-
  Subtract_52509 : Sum  Inputs=+-
  Subtract_6a2da : Sum  Inputs=+-
  Subtract_b1140 : Sum  Inputs=+-
  Subtract_b5aaa : Sum  Inputs=+-
  Subtract_d2889 : Sum  Inputs=+-
  Subtract_e5eb1 : Sum  Inputs=+-
  Blockout_d_psi_gq_SG_D_2_9dda3 : Outport
  wires:
  Constant_x_l_f750d/1 -> Product_b7555/2
  Constant_x_l_0becc/1 -> Product_bad74/2
  Constant_x_qd_976aa/1 -> Subtract_b1140/1
  Constant_x_l_74850/1 -> Product_de8f0/2
  Constant_x_qdd_840b2/1 -> Subtract_b5aaa/2
  Constant_-1_60b81/1 -> Product_d6121/1
  Constant_-1_ef641/1 -> Product_eecf6/1
  State_psi_gq_SG_D_2_262b6/1 -> Add_df759/1
  Constant_x_qdd_79456/1 -> Subtract_b1140/2
  Constant_x_qd_43aff/1 -> Subtract_b5aaa/1
  Constant_x_l_64566/1 -> Product_d6121/2
  Constant_x_l_8b370/1 -> Product_eecf6/2
  Product_d6121/1 -> Add_a8284/1
  Product_eecf6/1 -> Add_fa509/1
  Constant_x_l_6a069/1 -> Product_67582/2
  Constant_x_l_212c0/1 -> Product_9f606/2
  Constant_x_qd_e2fa8/1 -> Add_a8284/2
  Constant_x_qdd_f547d/1 -> Add_fa509/2
  Constant_-1_c26a6/1 -> Product_67582/1
  Constant_x_qd_c4800/1 -> Add_09fd3/2
  Constant_x_qdd_81909/1 -> Add_4f66c/2
  State_psi_gq_SG_D_2_5c0ba/1 -> Product_733a0/1
  Add_a8284/1 -> Divide_a8046/2
  Add_fa509/1 -> Product_733a0/2
  Constant_x_qd_8bff0/1 -> Subtract_37c15/2
  Product_67582/1 -> Add_ee4d9/1
  Constant_x_qd_7784c/1 -> Add_ee4d9/2
  State_psi_kq_SG_D_2_f72a7/1 -> Product_7d711/1
  Divide_8a6bf/1 -> Subtract_d2889/1
  Subtract_b1140/1 -> Product_7d711/2
  Product_733a0/1 -> Divide_8a6bf/1
  Add_ee4d9/1 -> Divide_8a6bf/2
  Add_434fc/1 -> Product_c1033/2
  Product_7d711/1 -> Divide_a8046/1
  Constant_-1_155a2/1 -> Product_9f606/1
  Divide_a8046/1 -> Subtract_d2889/2
  Constant_-1_54478/1 -> Product_b7555/1
  Constant_-1_0b5b8/1 -> Product_bad74/1
  Product_9f606/1 -> Add_ad1b5/1
  Constant_x_qdd_65e24/1 -> Subtract_25fd5/2
  Constant_x_qd_3cb96/1 -> Add_ad1b5/2
  Subtract_d2889/1 -> Add_434fc/1
  Constant_-1_fa415/1 -> Product_de8f0/1
  State_psi_q_SG_D_2_7c5c2/1 -> Add_434fc/2
  Product_b7555/1 -> Add_09fd3/1
  Product_bad74/1 -> Add_4f66c/1
  Constant_-1_b12ee/1 -> Product_32f08/1
  Product_c1033/1 -> Divide_ad28d/1
  Constant_x_l_a473e/1 -> Product_32f08/2
  Product_aec92/1 -> Add_2f5da/2
  Constant_x_qd_a1839/1 -> Subtract_25fd5/1
  Add_ad1b5/1 -> Product_c1033/1
  State_psi_gq_SG_D_2_708e2/1 -> Product_d6a36/1
  Add_09fd3/1 -> Divide_d6170/2
  Add_4f66c/1 -> Product_d6a36/2
  Product_32f08/1 -> Add_1216c/1
  Constant_x_qd_36ccd/1 -> Add_1216c/2
  State_psi_kq_SG_D_2_8a990/1 -> Product_094d9/1
  Subtract_25fd5/1 -> Product_094d9/2
  Divide_d6170/1 -> Subtract_52509/2
  State_psi_kq_SG_D_2_70141/1 -> Add_df759/2
  Product_094d9/1 -> Divide_d6170/1
  Constant_x_qdd_1828c/1 -> Divide_ad28d/2
  Product_d6a36/1 -> Divide_cb966/1
  Add_1216c/1 -> Divide_cb966/2
  Constant_-1_14cc3/1 -> Product_2238e/1
  Subtract_b5aaa/1 -> Product_2238e/2
  Add_df759/1 -> Subtract_6a2da/1
  Divide_ad28d/1 -> Subtract_6a2da/2
  Product_de8f0/1 -> Add_fca1a/1
  Constant_x_qd_889c4/1 -> Add_fca1a/2
  Divide_cb966/1 -> Subtract_52509/1
  Product_2238e/1 -> Product_1c512/1
  Subtract_6a2da/1 -> Product_1c512/2
  Add_fca1a/1 -> Power_78b4e/1
  Constant_2.0_27ef5/1 -> Power_78b4e/2
  Subtract_52509/1 -> Add_c990e/1
  State_psi_q_SG_D_2_071fc/1 -> Add_c990e/2
  Product_1c512/1 -> Divide_3e593/1
  Power_78b4e/1 -> Divide_3e593/2
  Add_c990e/1 -> Divide_4fc6b/1
  Constant_x_qdd_a8df6/1 -> Divide_4fc6b/2
  Constant_x_q_9f5a2/1 -> Subtract_37c15/1
  Divide_3e593/1 -> Subtract_e5eb1/1
  Divide_4fc6b/1 -> Subtract_e5eb1/2
  Divide_f8b90/1 -> Blockout_d_psi_gq_SG_D_2_9dda3/1
  Constant_-1_3830c/1 -> Product_c5194/1
  State_psi_gq_SG_D_2_6e627/1 -> Product_c5194/2
  Subtract_37c15/1 -> Product_aec92/1
  Subtract_e5eb1/1 -> Product_aec92/2
  Product_c5194/1 -> Add_2f5da/1
  Add_2f5da/1 -> Divide_f8b90/1
  Constant_T_qd_93225/1 -> Divide_f8b90/2

== system case8/SG_D_2/d_psi_kq_SG_D_2_block ==
  note: d_psi_kq_SG_D_2 in case8
      | $-\frac{\psi _{\mathrm{gq},\mathrm{SG},D,2}+\psi _{\mathrm{kq},\mathrm{SG},D,2}+\frac{\left(x_{l}-x_{\mathrm{qd}}\right)\,\left(\psi _{q,\mathrm{SG},D,2}+\frac{\psi _{\mathrm{gq},\mathrm{SG},D,2}\,\left(x_{l}-x_{\mathrm{qdd}}\right)}{x_{l}-x_{\mathrm{qd}}}+\frac{\psi _{\mathrm{kq},\mathrm{SG},D,2}\,\left(x_{\mathrm{qd}}-x_{\mathrm{qdd}}\right)}{x_{l}-x_{\mathrm{qd}}}\right)}{x_{\mathrm{qdd}}}}{T_{\mathrm{qdd}}}$
      | Automatically generated on 2025-10-31 19:29:52 .
  State_psi_gq_SG_D_2_71331 : Inport
  State_psi_kq_SG_D_2_cb04f : Inport  Port=2
  State_psi_gq_SG_D_2_5efea : Inport  Port=3
  State_psi_kq_SG_D_2_ff070 : Inport  Port=4
  State_psi_q_SG_D_2_e3912 : Inport  Port=5
  Add_5cc98 : Sum
  Add_73138 : Sum
  Add_aae72 : Sum
  Add_c9773 : Sum
  Add_cb050 : Sum
  Add_d79ce : Sum
  Constant_-1_48b0e : Constant  Value=-1
  Constant_-1_96575 : Constant  Value=-1
  Constant_-1_a96f8 : Constant  Value=-1
  Constant_-1_ad55f : Constant  Value=-1
  Constant_-1_e8813 : Constant  Value=-1
  Constant_T_qdd_68214 : Constant  Value=T_qdd
  Constant_x_l_503d1 : Constant  Value=x_l
  Constant_x_l_849b4 : Constant  Value=x_l
  Constant_x_l_99a7a : Constant  Value=x_l
  Constant_x_l_a58a2 : Constant  Value=x_l
  Constant_x_qd_01a68 : Constant  Value=x_qd
  Constant_x_qd_1bb99 : Constant  Value=x_qd
  Constant_x_qd_2946d : Constant  Value=x_qd
  Constant_x_qd_c4114 : Constant  Value=x_qd
  Constant_x_qdd_04784 : Constant  Value=x_qdd
  Constant_x_qdd_7d270 : Constant  Value=x_qdd
  Constant_x_qdd_e41d7 : Constant  Value=x_qdd
  Divide_7b5df : Product  Inputs=*/
  Divide_97e00 : Product  Inputs=*/
  Divide_9d864 : Product  Inputs=*/
  Divide_bf659 : Product  Inputs=*/
  Product_0ab54 : Product
  Product_0bb2d : Product
  Product_39b82 : Product
  Product_3d284 : Product
  Product_5dffe : Product
  Product_6433a : Product
  Product_e422b : Product
  Product_f57a7 : Product
  Subtract_4a934 : Sum  Inputs=+-
  Subtract_b1397 : Sum  Inputs=+-
  Subtract_e2b6c : Sum  Inputs=+-
  Blockout_d_psi_kq_SG_D_2_314e9 : Outport
  wires:
  State_psi_kq_SG_D_2_cb04f/1 -> Subtract_e2b6c/2
  Constant_-1_48b0e/1 -> Product_e422b/1
  Constant_-1_ad55f/1 -> Product_3d284/1
  Constant_x_l_a58a2/1 -> Product_3d284/2
  Constant_x_qdd_e41d7/1 -> Add_5cc98/2
  Constant_x_l_99a7a/1 -> Product_e422b/2
  Constant_x_qd_01a68/1 -> Subtract_4a934/1
  Constant_T_qdd_68214/1 -> Divide_bf659/2
  Constant_-1_e8813/1 -> Product_5dffe/1
  Product_3d284/1 -> Add_5cc98/1
  Constant_x_qdd_04784/1 -> Subtract_4a934/2
  Constant_x_l_503d1/1 -> Product_5dffe/2
  Divide_bf659/1 -> Blockout_d_psi_kq_SG_D_2_314e9/1
  State_psi_gq_SG_D_2_5efea/1 -> Product_0bb2d/1
  Add_5cc98/1 -> Product_0bb2d/2
  Product_e422b/1 -> Add_aae72/1
  Constant_x_qd_c4114/1 -> Add_aae72/2
  Product_6433a/1 -> Divide_7b5df/1
  State_psi_kq_SG_D_2_ff070/1 -> Product_39b82/1
  Subtract_4a934/1 -> Product_39b82/2
  Product_5dffe/1 -> Add_73138/1
  Constant_x_qd_1bb99/1 -> Add_73138/2
  Product_39b82/1 -> Divide_9d864/1
  Product_0bb2d/1 -> Divide_97e00/1
  Add_aae72/1 -> Divide_97e00/2
  Add_73138/1 -> Divide_9d864/2
  State_psi_q_SG_D_2_e3912/1 -> Add_c9773/2
  Constant_-1_96575/1 -> Product_0ab54/1
  Constant_x_l_849b4/1 -> Product_0ab54/2
  Divide_97e00/1 -> Subtract_b1397/1
  Divide_9d864/1 -> Subtract_b1397/2
  Product_0ab54/1 -> Add_cb050/1
  Constant_x_qd_2946d/1 -> Add_cb050/2
  Subtract_b1397/1 -> Add_c9773/1
  Constant_x_qdd_7d270/1 -> Divide_7b5df/2
  Constant_-1_a96f8/1 -> Product_f57a7/1
  State_psi_gq_SG_D_2_71331/1 -> Product_f57a7/2
  Add_cb050/1 -> Product_6433a/1
  Add_c9773/1 -> Product_6433a/2
  Product_f57a7/1 -> Subtract_e2b6c/1
  Subtract_e2b6c/1 -> Add_d79ce/1
  Divide_7b5df/1 -> Add_d79ce/2
  Add_d79ce/1 -> Divide_bf659/1

== system case8/SG_D_2/d_psi_q_SG_D_2_block ==
  note: d_psi_q_SG_D_2 in case8
      | $2\,\pi \,f_{0}\,\left(v_{d,\mathrm{SG},D,2}\,\cos\left(\theta _{\mathrm{SG},D,2}\right)+v_{q,\mathrm{SG},D,2}\,\sin\left(\theta _{\mathrm{SG},D,2}\right)-\frac{R_{a}\,\left(\psi _{q,\mathrm{SG},D,2}+\frac{\psi _{\mathrm{gq},\mathrm{SG},D,2}\,\left(x_{l}-x_{\mathrm{qdd}}\right)}{x_{l}-x_{\mathrm{qd}}}+\frac{\psi _{\mathrm{kq},\mathrm{SG},D,2}\,\left(x_{\mathrm{qd}}-x_{\mathrm{qdd}}\right)}{x_{l}-x_{\mathrm{qd}}}\right)}{x_{\mathrm{qdd}}}-\frac{\psi _{d,\mathrm{SG},D,2}\,w_{\mathrm{SG},D,2}}{2\,f_{0}\,\pi }\right)$
      | Automatically generated on 2025-10-31 19:29:47 .
  State_psi_gq_SG_D_2_5ef83 : Inport
  State_psi_kq_SG_D_2_f0515 : Inport  Port=2
  State_psi_q_SG_D_2_4fbbc : Inport  Port=3
  Input_v_d_SG_D_2_d12f5 : Inport  Port=4
  State_theta_SG_D_2_e72a3 : Inport  Port=5
  Input_v_q_SG_D_2_08eca : Inport  Port=6
  State_theta_SG_D_2_47452 : Inport  Port=7
  State_psi_d_SG_D_2_64c51 : Inport  Port=8
  State_w_SG_D_2_341ca : Inport  Port=9
  Add_27575 : Sum
  Add_8fe18 : Sum
  Add_bfee9 : Sum
  Add_f2802 : Sum
  Add_ffc6f : Sum
  Constant_-1_62a2d : Constant  Value=-1
  Constant_-1_6559a : Constant  Value=-1
  Constant_-1_8ac1d : Constant  Value=-1
  Constant_-2.0_b2469 : Constant  Value=-2.0
  Constant_2.0_2466a : Constant  Value=2.0
  Constant_R_a_47e98 : Constant  Value=R_a
  Constant_f0_9713d : Constant  Value=f0
  Constant_f0_cd56b : Constant  Value=f0
  Constant_pi_356fc : Constant  Value=pi
  Constant_pi_40a79 : Constant  Value=pi
  Constant_x_l_34939 : Constant  Value=x_l
  Constant_x_l_c4449 : Constant  Value=x_l
  Constant_x_l_eb517 : Constant  Value=x_l
  Constant_x_qd_07b2e : Constant  Value=x_qd
  Constant_x_qd_0fb8f : Constant  Value=x_qd
  Constant_x_qd_1426f : Constant  Value=x_qd
  Constant_x_qdd_35a04 : Constant  Value=x_qdd
  Constant_x_qdd_4e846 : Constant  Value=x_qdd
  Constant_x_qdd_a1503 : Constant  Value=x_qdd
  Divide_21611 : Product  Inputs=*/
  Divide_2db25 : Product  Inputs=*/
  Divide_51057 : Product  Inputs=*/
  Divide_a652c : Product  Inputs=*/
  MathFunc_cos_7f82a : Trigonometry  Operator=cos
  MathFunc_sin_57505 : Trigonometry
  Product_116ea : Product
  Product_19730 : Product
  Product_1f0bd : Product
  Product_20595 : Product
  Product_38024 : Product
  Product_50ee5 : Product
  Product_5330d : Product
  Product_6333e : Product
  Product_642ff : Product
  Product_69dbc : Product
  Product_78f90 : Product
  Product_7da29 : Product
  Product_b7c7d : Product
  Product_bbe65 : Product
  Subtract_02e32 : Sum  Inputs=+-
  Subtract_1da1a : Sum  Inputs=+-
  Subtract_55c59 : Sum  Inputs=+-
  Subtract_8f1b2 : Sum  Inputs=+-
  Blockout_d_psi_q_SG_D_2_ca292 : Outport
  wires:
  Constant_x_qdd_35a04/1 -> Subtract_02e32/2
  Constant_x_l_34939/1 -> Product_1f0bd/2
  Constant_-1_8ac1d/1 -> Product_19730/1
  Constant_x_l_eb517/1 -> Product_19730/2
  Product_19730/1 -> Add_27575/1
  Constant_pi_40a79/1 -> Product_116ea/2
  State_psi_gq_SG_D_2_5ef83/1 -> Product_6333e/1
  Constant_x_l_c4449/1 -> Product_5330d/2
  State_w_SG_D_2_341ca/1 -> Product_38024/2
  Constant_x_qd_0fb8f/1 -> Add_8fe18/2
  Constant_x_qdd_a1503/1 -> Add_27575/2
  Constant_2.0_2466a/1 -> Product_116ea/1
  Constant_-1_6559a/1 -> Product_5330d/1
  Constant_x_qd_07b2e/1 -> Subtract_02e32/1
  Constant_-1_62a2d/1 -> Product_1f0bd/1
  State_psi_q_SG_D_2_4fbbc/1 -> Add_ffc6f/2
  Add_27575/1 -> Product_6333e/2
  Product_116ea/1 -> Product_b7c7d/1
  Product_5330d/1 -> Add_f2802/1
  Constant_pi_356fc/1 -> Product_50ee5/2
  Constant_f0_cd56b/1 -> Product_b7c7d/2
  Constant_x_qd_1426f/1 -> Add_f2802/2
  State_psi_kq_SG_D_2_f0515/1 -> Product_20595/1
  Subtract_02e32/1 -> Product_20595/2
  Product_1f0bd/1 -> Add_8fe18/1
  Input_v_q_SG_D_2_08eca/1 -> Product_642ff/1
  Product_6333e/1 -> Divide_2db25/1
  Product_b7c7d/1 -> Divide_21611/2
  Add_f2802/1 -> Divide_2db25/2
  Product_20595/1 -> Divide_a652c/1
  Add_8fe18/1 -> Divide_a652c/2
  Divide_2db25/1 -> Subtract_1da1a/1
  State_theta_SG_D_2_e72a3/1 -> MathFunc_cos_7f82a/1
  Divide_a652c/1 -> Subtract_1da1a/2
  Subtract_1da1a/1 -> Add_ffc6f/1
  MathFunc_cos_7f82a/1 -> Product_bbe65/2
  Constant_R_a_47e98/1 -> Product_7da29/1
  Add_ffc6f/1 -> Product_7da29/2
  State_theta_SG_D_2_47452/1 -> MathFunc_sin_57505/1
  Product_7da29/1 -> Divide_51057/1
  Product_50ee5/1 -> Product_69dbc/1
  Product_642ff/1 -> Subtract_8f1b2/2
  Constant_x_qdd_4e846/1 -> Divide_51057/2
  Input_v_d_SG_D_2_d12f5/1 -> Product_bbe65/1
  Add_bfee9/1 -> Product_78f90/2
  Divide_51057/1 -> Subtract_55c59/1
  Product_bbe65/1 -> Subtract_55c59/2
  MathFunc_sin_57505/1 -> Product_642ff/2
  Product_78f90/1 -> Blockout_d_psi_q_SG_D_2_ca292/1
  State_psi_d_SG_D_2_64c51/1 -> Product_38024/1
  Constant_-2.0_b2469/1 -> Product_50ee5/1
  Product_69dbc/1 -> Product_78f90/1
  Subtract_55c59/1 -> Subtract_8f1b2/1
  Product_38024/1 -> Divide_21611/1
  Constant_f0_9713d/1 -> Product_69dbc/2
  Subtract_8f1b2/1 -> Add_bfee9/1
  Divide_21611/1 -> Add_bfee9/2

== system case8/SG_D_2/d_theta_SG_D_2_block ==
  note: d_theta_SG_D_2 in case8
      | $w_{\mathrm{SG},D,2}-2\,\pi \,f_{0}$
      | Automatically generated on 2025-10-31 19:29:53 .
  State_w_SG_D_2_7bd31 : Inport
  Add_7a9ad : Sum
  Constant_-2.0_bce4d : Constant  Value=-2.0
  Constant_f0_5facc : Constant  Value=f0
  Constant_pi_6a525 : Constant  Value=pi
  Product_ee788 : Product
  Product_fed01 : Product
  Blockout_d_theta_SG_D_2_25192 : Outport
  wires:
  Constant_-2.0_bce4d/1 -> Product_ee788/1
  Constant_pi_6a525/1 -> Product_ee788/2
  Add_7a9ad/1 -> Blockout_d_theta_SG_D_2_25192/1
  Product_ee788/1 -> Product_fed01/1
  Constant_f0_5facc/1 -> Product_fed01/2
  Product_fed01/1 -> Add_7a9ad/1
  State_w_SG_D_2_7bd31/1 -> Add_7a9ad/2
